simulink model "MalaksModel"  (R2022a)
settings: Solver=FixedStepAuto  StartTime=0.0  StopTime=10  FixedStep=0.001  MaxStep=1  MinStep=5e-4  RelTol=1e-3  EnableMultiTasking=on
values from neighbouring files (symbols this model uses):
  B = 0.00416    [Allan_Param.m]
  b1 = Bf/2    (= 0.776)    [model_10DOF_revised.m]
  b2 = b1    (= 0.776)    [model_10DOF_revised.m]
  b3 = Br/2    (= 0.78)    [model_10DOF_revised.m]
  b4 = b3    (= 0.78)    [model_10DOF_revised.m]
  Beq = 0.0001    [model_10DOF_revised.m]
  Bf = 1.552    [model_10DOF_revised.m]
  cs1 = 4500    [model_10DOF_revised.m]
  cs2 = 4500    [model_10DOF_revised.m]
  cs3 = 11207    [model_10DOF_revised.m]
  dpc = h-hzpc    (= 0.4878144918)    [model_10DOF_revised.m]
  drc = h-hzrc    (= 0.4878144918)    [model_10DOF_revised.m]
  Fs = 100    [Allan_Param.m]
  g = 9.81    [model_10DOF_revised.m]
  hzpc = 0.05    [model_10DOF_revised.m]
  hzrc = 0.05    [model_10DOF_revised.m]
  Ix = 233.072773102 + m*drc^2    (= 616.009936849)    [model_10DOF_revised.m]
  Ix_Iy = Ix -Iy    (= -852.927226898)    [model_10DOF_revised.m]
  Iy = 1086 + m*dpc^2    (= 1468.93716375)    [model_10DOF_revised.m]
  Iy_Iz = Iy -Iz    (= 281.937163747)    [model_10DOF_revised.m]
  Iz = 1187    [model_10DOF_revised.m]
  Iz_Ix = Iz -Ix    (= 570.990063151)    [model_10DOF_revised.m]
  Jeq = 0.00025    [model_10DOF_revised.m]
  K = 1.4e-3    (= 0.0014)    [Allan_Param.m]
  Ka = 0.05    [model_10DOF_revised.m]
  Ke = 0.168    [model_10DOF_revised.m]
  L = 2.72    [model_10DOF_revised.m]
  l1 = 1.12695753    [model_10DOF_revised.m]
  l2 = L-l1    (= 1.59304247)    [model_10DOF_revised.m]
  Leq = 1.5e-3    (= 0.0015)    [model_10DOF_revised.m]
  m = MT-(muf+mur)    (= 1609.23)    [model_10DOF_revised.m]
  mu = 0.8    [model_10DOF_revised.m]
  mu1 = muf/2    (= 49.5)    [model_10DOF_revised.m]
  mu2 = mu1    (= 49.5)    [model_10DOF_revised.m]
  mu3 = mur/2    (= 42)    [model_10DOF_revised.m]
  mu4 = mu3    (= 42)    [model_10DOF_revised.m]
  N = 0.00166667    [Allan_Param.m]
  radius = 40    [path1.m]
  Req = 0.5    [model_10DOF_revised.m]
  ro = 0    [Input.m]
  sw_delta_f = 1    [Input.m]
  Tc = 32    [Allan_Param.m]
  THETAo = 0    [Input.m]
  tpo = cp/6    (= 0.0333333333333)    [Input.m]
  vxo = 10    [Input.m]
  vyo = 0    [Input.m]
  Ws1 = (l2*Ws)/(2*L)    (= 4622.91152767)    [model_10DOF_revised.m]
  x = 0:1:200    [look_ahead.m]    (also in path1.m = x(:))
  Xo = 0    [Input.m]
  y = l_des    [look_ahead.m]    (also in path1.m = zeros(size(x)))
  Yo = 0    [Input.m]
  zu1_0 = -W1/k1t    (= -0.0255425326383)    [model_10DOF_revised.m]
  zu2_0 = -W2/k2t    (= -0.0255425326383)    [model_10DOF_revised.m]
  zu3_0 = -W3/k3t    (= -0.0184119081117)    [model_10DOF_revised.m]
  zu4_0 = -W4/k4t    (= -0.0184119081117)    [model_10DOF_revised.m]
undefined symbols (not defined in the file or in its folder): sw_phi, sw_psi, sw_theta, sw_x, sw_y, sw_zs, sw_zu1, sw_zu2, sw_zu3, sw_zu4
libraries: slpidlib x6, ec_arm_cortex_a_lib x1
(part 1 of 2)
settings Model: Creator=Mohammad Almalak  LastModifiedBy=Mohammad Almalak
settings SolverCC: MaxConsecutiveMinStep=10  PositivePriorityOrder=on
settings OptimizationCC: GainParamInheritBuiltInType=on  DefaultUnderspecifiedDataType=single  EnhancedBackFolding=on  PassReuseOutputArgsAs=Individual arguments  ZeroExternalMemoryAtStartup=off  ZeroInternalMemoryAtStartup=off  MaxStackSize=64  OptimizeBlockOrder=speed  DifferentSizesBufferReuse=on  OptimizationCustomize=off  EfficientTunableParamExpr=on
settings DebuggingCC: ParameterTunabilityLossMsg=error
settings HardwareCC: ProdBitPerPointer=32  ProdBitPerSizeT=32  ProdBitPerPtrDiffT=32  ProdLargestAtomicInteger=Long  ProdLargestAtomicFloat=Double  ProdWordSize=32  ProdHWDeviceType=ARM Compatible->ARM Cortex  TargetBitPerPointer=64  TargetBitPerSizeT=64  TargetBitPerPtrDiffT=64  TargetLongLongMode=on  TargetIntDivRoundTo=Zero  TargetEndianess=LittleEndian  TargetWordSize=64  TargetHWDeviceType=MATLAB Host
settings ModelReferenceCC: ModelReferenceNumInstancesAllowed=Single  ModelReferenceMinAlgLoopOccurrences=on
settings SFSimCC: MATLABDynamicMemAlloc=off
settings RTWCC: SystemTargetFile=ert.tlc  HardwareBoard=BeagleBone Black  TLCOptions="-aInlineSetEventsForThisBaseRateFcn=TLC_FALSE -aSuppressMultiTaskScheduler=TLC_FALSE  -aRateBasedStepFcn=0"  TemplateMakefile=ert_default_tmf  GenerateReport=on  RTWVerbose=off  Toolchain=Linaro Toolchain v4.8  BuildConfiguration=Faster Runs
settings CodeAppCC: ForceParamTrailComments=on  IgnoreCustomStorageClasses=off  MaxIdLength=255  OperatorAnnotations=on  SimulinkDataObjDesc=on  SFDataObjDesc=on  InsertBlockDesc=on
settings ERTTargetCC: SupportContinuousTime=on

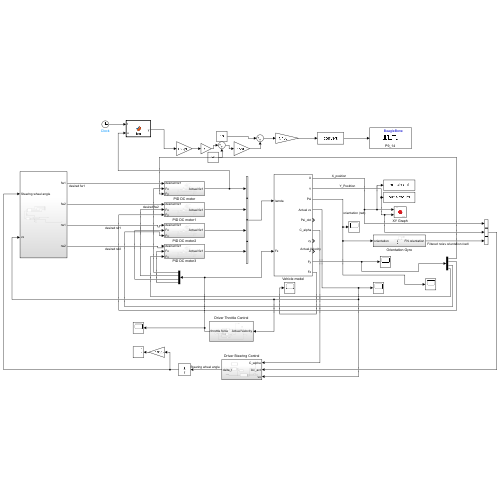
[thumbnail: Simulink's stored preview of the top-level diagram]
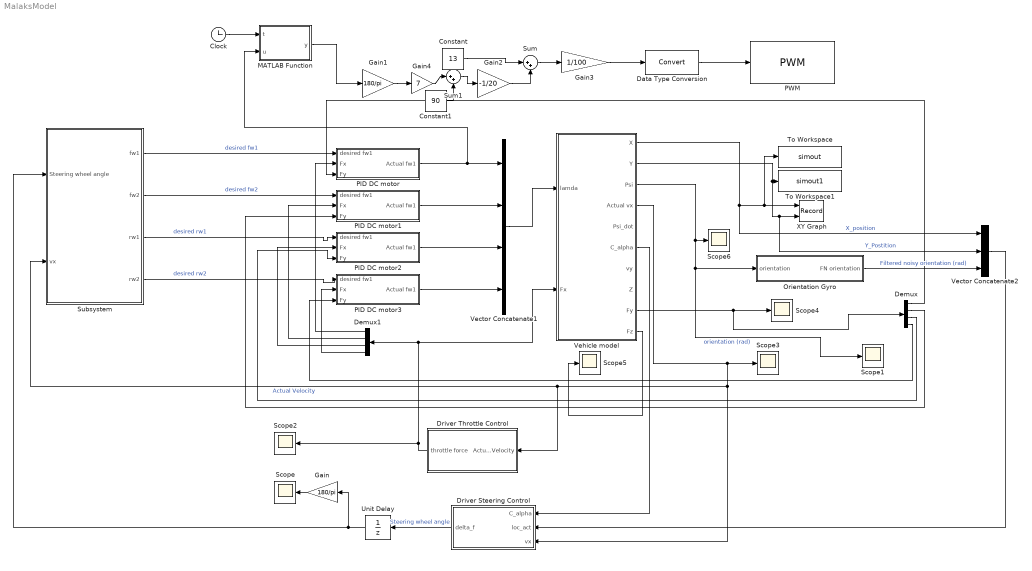
== system MalaksModel ==
  Clock : Clock
  Constant : Constant  Value=13
  Constant1 : Constant  Value=90
  Data Type Conversion : DataTypeConversion  SaturateOnIntegerOverflow=off  RndMeth=Floor
  Demux : Demux
  Demux1 : Demux
  Driver Steering Control : Subsystem
  Driver Throttle Control : Subsystem
  Gain : Gain  Gain=180/pi
  Gain1 : Gain  Gain=180/pi
  Gain2 : Gain  Gain=-1/20
  Gain3 : Gain  Gain=1/100
  Gain4 : Gain  Gain=7
  MATLAB Function : MATLAB Function  TreatAsAtomicUnit=on
  Orientation Gyro : Subsystem
  PID DC motor : Subsystem
  PID DC motor1 : Subsystem
  PID DC motor2 : Subsystem
  PID DC motor3 : Subsystem
  PWM : ec_arm_cortex_a_lib/PWM  board=BeagleBone Black  pin=P9_14  frequency=50  polarity=Positive  blockPlatform=BeagleBone
      settings: SourceProductBaseCode=ECCORTEXA
  Scope{,1..6} (7 alike) : Scope
  Subsystem : Subsystem
  Sum : Sum  Inputs=|++
  Sum1 : Sum  Inputs=|++
  To Workspace : ToWorkspace  VariableName=simout  SaveFormat=Timeseries  SampleTime=-1
  To Workspace1 : ToWorkspace  VariableName=simout1  SaveFormat=Timeseries  SampleTime=-1
  Unit Delay : UnitDelay  SampleTime=-1  HasFrameUpgradeWarning=on
  Vector Concatenate1 : Concatenate  NumInputs=4  ConcatenateDimension=2
  Vector Concatenate2 : Concatenate  NumInputs=3
  Vehicle model : Subsystem
  XY Graph : Record  FileSettingsInternal="{\"entries\":[{\"content\":{\"excelSettings\":{\"content\":{},\"type\":\"Streamout.ExcelSettings\"}},\"type\":\"Streamout.FileSettingStorage\",\"uuid\":\"fef33843-d556-4eb6-a8ea-e7493e2dd152\"}],\"packageUris\":[\"http://schema.mathworks.com/mf0/streamout_blocks/R2020a\"],\"version\":\"1.0\"}"  Layout=[1 1]  SignalsInternal="{\"entries\":[{\"content\":{\"signals\":[{\"content\":{\"blockPath\":[\"MalaksModel/XY Graph\"],\"channel\":[],\"dimensions\":[1],\"domain\":\"MalaksModel/XY Graph\",\"lineColor\":\"#a2142f\",\"plots\":[1],\"port\":1,\"sid\":[\"\"],\"signalID\":362,\"signalName\":\"X_position\"},\"type\":\"RecordBlkView.Signal\",\"uuid\":\"be4ed4d4-a0e0-4c05-83f8-aa9f8cd4aeaf\"},{\"content\":{\"blockPath\":[\"MalaksModel/XY Graph\"],\"channel\":[],\"dimensions\":[1],\"domain\":\"MalaksModel/XY Graph\",\"lineColor\":\"#139fff\",\"plots\":[1],\"port\":2,\"sid\":[\"\"],\"signalID\":366,\"signalName\":\"Y_Postition\"},\"type\":\"RecordBlkView.Signal\",\"uuid\":\"7f74b197-2333-44af-aabe-7eaf48b827cd\"}]},\"type\":\"RecordBlkView.InputSignals\",\"uuid\":\"3425b8f1-97a8-43f9-8de6-0b3d5bc8f21d\"}],\"packageUris\":[\"http://schema.mathworks.com/mf0/streamout_blocks/R2020a\"],\"version\":\"1.0\"}"  VisualizationBindings="{\"xyplotplugin\":{\"info\":[{\"series\":[{\"bindingParametersList\":[{\"parameter\":\"X-Axis\",\"signalID\":362,\"signalName\":\"X_position\"},{\"parameter\":\"Y-Axis\",\"signalID\":366,\"signalName\":\"Y_Postition\"}],\"seriesID\":32300}],\"subplotID\":1}]}}"  CompatibilityTag=XY
  wires:
  Vector Concatenate1/1 -> Vehicle model/1(lamda)
  Vehicle model/3(Psi) -> Scope6/1, Orientation Gyro/1(orientation), Scope1/1  "orientation (rad)"
  Vehicle model/2(Y) -> Vector Concatenate2/2, XY Graph/2, To Workspace1/1  "Y_Postition"
  Vehicle model/1(X) -> Vector Concatenate2/1, To Workspace/1, XY Graph/1  "X_position"
  Vehicle model/4(Actual vx) -> Scope3/1, Driver Steering Control/3(vx), Subsystem/2(vx), Driver Throttle Control/1(Actual Velocity)  "Actual Velocity"
  Vector Concatenate2/1 -> Driver Steering Control/2(loc_act)
  Driver Steering Control/1(delta_f) -> Unit Delay/1  "Steering wheel angle"
  Subsystem/2(fw2) -> PID DC motor1/1(desired fw1)  "desired fw2"
  Subsystem/3(rw1) -> PID DC motor2/1(desired fw1)  "desired rw1"
  Gain/1 -> Scope/1
  Subsystem/4(rw2) -> PID DC motor3/1(desired fw1)  "desired rw2"
  Subsystem/1(fw1) -> PID DC motor/1(desired fw1)  "desired fw1"
  PID DC motor1/1(Actual fw1) -> Vector Concatenate1/2
  PID DC motor2/1(Actual fw1) -> Vector Concatenate1/3
  PID DC motor3/1(Actual fw1) -> Vector Concatenate1/4
  Driver Throttle Control/1(throttle force) -> Scope2/1, Vehicle model/2(Fx), Demux1/1
  Vehicle model/9(Fy) -> Demux/1, Scope4/1
  Demux/1 -> PID DC motor/3(Fy)
  Demux1/1 -> PID DC motor/2(Fx)
  Orientation Gyro/1(FN orientation) -> Vector Concatenate2/3  "Filtered noisy orientation (rad)"
  Demux1/2 -> PID DC motor1/2(Fx)
  Demux1/3 -> PID DC motor2/2(Fx)
  Demux1/4 -> PID DC motor3/2(Fx)
  Demux/2 -> PID DC motor1/3(Fy)
  Demux/3 -> PID DC motor2/3(Fy)
  Demux/4 -> PID DC motor3/3(Fy)
  Vehicle model/10(Fz) -> Scope5/1
  Gain1/1 -> Gain4/1
  Gain2/1 -> Sum/2
  Constant/1 -> Sum/1
  Sum/1 -> Gain3/1
  Data Type Conversion/1 -> PWM/1
  Gain3/1 -> Data Type Conversion/1
  PID DC motor/1(Actual fw1) -> MATLAB Function/2(u), Vector Concatenate1/1
  Vehicle model/6(C_alpha) -> Driver Steering Control/1(C_alpha)
  Unit Delay/1 -> Gain/1, Subsystem/1(Steering wheel angle)
  Gain4/1 -> Sum1/1
  Sum1/1 -> Gain2/1
  Constant1/1 -> Sum1/2
  Clock/1 -> MATLAB Function/1(t)
  MATLAB Function/1(y) -> Gain1/1

== system MalaksModel/Driver Steering Control ==
  C_alpha : Inport  OutDataTypeStr=double
  loc_act : Inport  Port=2  OutDataTypeStr=double
  vx : Inport  Port=3  OutDataTypeStr=double
  FWS Controller : MATLAB Function  TreatAsAtomicUnit=on
  From Workspace : FromWorkspace  VariableName=delta_f
  Subsystem : Subsystem
  Subsystem1 : Subsystem
  delta_f : Outport  OutDataTypeStr=double
  wires:
  FWS Controller/1(ackerman) -> delta_f/1, Subsystem/2(ackerman)
  loc_act/1 -> FWS Controller/1(loc_act)
  C_alpha/1 -> FWS Controller/3(C_alpha)
  From Workspace/1 -> Subsystem/1(In2)
  vx/1 -> FWS Controller/2(vx)

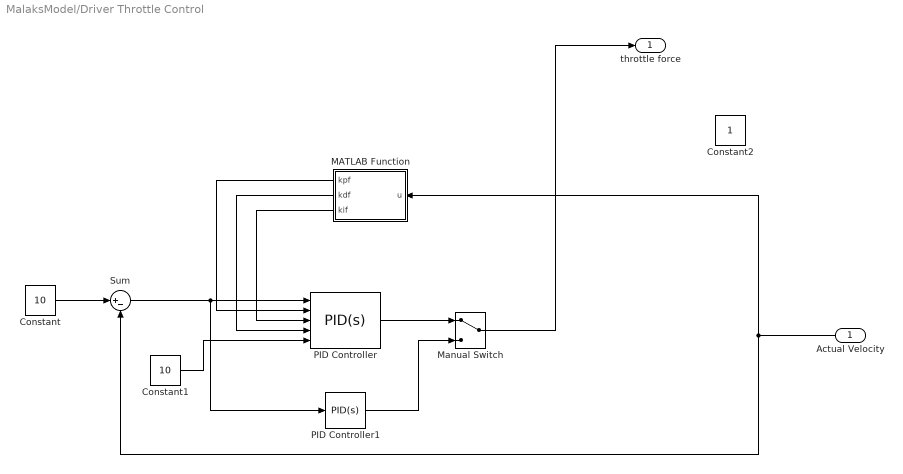
== system MalaksModel/Driver Throttle Control ==
  Actual Velocity : Inport  OutDataTypeStr=double
  Constant : Constant  Value=10
  Constant1 : Constant  Value=10
  Constant2 : Constant
  MATLAB Function : MATLAB Function  TreatAsAtomicUnit=on
  Manual Switch : ManualSwitch
  PID Controller : slpidlib/PID Controller  Controller=PID  Form=Parallel  TimeDomain=Continuous-time  UseExternalTs=off  SampleTime=-1  IntegratorMethod=Forward Euler  FilterMethod=Forward Euler  ControllerParametersSource=external  P=1  I=1  UseKiTs=off  D=0  N=100  UseFilter=on  TunerSelectOption=Transfer Function Based (PID Tuner App)  InitialConditionSource=internal  InitialConditionForIntegrator=0  InitialConditionForFilter=0  DifferentiatorICPrevScaledInput=0  ExternalReset=none  TrackingMode=off  Kt=1  LimitOutput=off  SatLimitsSource=internal  UpperSaturationLimit=inf  LowerSaturationLimit=-inf  LinearizeAsGain=on  AntiWindupMode=none  Kb=1  POutMin=[]  POutMax=[]  IOutMin=[]  IOutMax=[]  DOutMin=[]  DOutMax=[]  NOutMin=[]  NOutMax=[]  SumOutMin=[]  SumOutMax=[]  SaturationOutMin=[]  SaturationOutMax=[]  PParamMin=[]  PParamMax=[]  IParamMin=[]  IParamMax=[]  DParamMin=[]  DParamMax=[]  NParamMin=[]  NParamMax=[]  KbParamMin=[]  KbParamMax=[]  KtParamMin=[]  KtParamMax=[]  KbOutMin=[]  KbOutMax=[]  KtOutMin=[]  KtOutMax=[]  IntegratorOutMin=[]  IntegratorOutMax=[]  FilterOutMin=[]  FilterOutMax=[]  SumI1OutMin=[]  SumI1OutMax=[]  SumI2OutMin=[]  SumI2OutMax=[]  SumI3OutMin=[]  SumI3OutMax=[]  SumI4OutMin=[]  SumI4OutMax=[]  SumDOutMin=[]  SumDOutMax=[]  DifferentiatorOutMin=[]  DifferentiatorOutMax=[]  FilterDiffOutCoefMin=[]  FilterDiffOutCoefMax=[]  ReciprocalOutMin=[]  ReciprocalOutMax=[]  SumDenOutMin=[]  SumDenOutMax=[]  SumNumOutMin=[]  SumNumOutMax=[]  DivideOutMin=[]  DivideOutMax=[]  UdiffTsProdOutMin=[]  UdiffTsProdOutMax=[]  NTsProdOutMin=[]  NTsProdOutMax=[]  UintegralTsProdOutMin=[]  UintegralTsProdOutMax=[]  UngainTsProdOutMin=[]  UngainTsProdOutMax=[]  IntegratorContinuousStateAttributes=''  IntegratorStateMustResolveToSignalObject=off  IntegratorRTWStateStorageClass=Auto  FilterContinuousStateAttributes=''  FilterStateMustResolveToSignalObject=off  FilterRTWStateStorageClass=Auto  ParallelPVariant=ExternalParameters  IdealPVariant=Disabled  IVariant=ExternalParameters  DVariant=ExternalParameters  IntegratorVariant=Continuous  SatVariant=Disabled  AWVariant=Passthrough  PCopyVariant=Disabled  TRVariant=Disabled  FdbkBlocksVariant=Forward  IdealPFdbkVariant=Disabled  SatFdbkVariant=Disabled  DerivativeFilterVariant=ContFilter  NVariant=ExternalParameters  NCopyVariant=Disabled  FilterICVariant=InternalICsFilter  IntegratorICVariant=InternalICs  ExternalResetVariant=Disabled  TRSumVariant=Passthrough  SumFdbkVariant=Disabled  SumVariant=Sum_PID  TsampFilterVariant=InternalTs  TsampNgainVariant=Passthrough  TsampIntegralVariant=Passthrough  ExternalSaturationOutDataTypeStr=Inherit: Same as second input  aMode=0
  PID Controller1 : slpidlib/PID Controller  Controller=PID  Form=Parallel  TimeDomain=Continuous-time  UseExternalTs=off  SampleTime=-1  IntegratorMethod=Forward Euler  FilterMethod=Forward Euler  ControllerParametersSource=internal  P=830.015869772746  I=316.552153422139  UseKiTs=off  D=9.58388407210146  N=238.770606857548  UseFilter=on  TunerSelectOption=Transfer Function Based (PID Tuner App)  InitialConditionSource=internal  InitialConditionForIntegrator=0  InitialConditionForFilter=0  DifferentiatorICPrevScaledInput=0  ExternalReset=none  TrackingMode=off  Kt=1  LimitOutput=off  SatLimitsSource=internal  UpperSaturationLimit=inf  LowerSaturationLimit=-inf  LinearizeAsGain=on  AntiWindupMode=none  Kb=1  POutMin=[]  POutMax=[]  IOutMin=[]  IOutMax=[]  DOutMin=[]  DOutMax=[]  NOutMin=[]  NOutMax=[]  SumOutMin=[]  SumOutMax=[]  SaturationOutMin=[]  SaturationOutMax=[]  PParamMin=[]  PParamMax=[]  IParamMin=[]  IParamMax=[]  DParamMin=[]  DParamMax=[]  NParamMin=[]  NParamMax=[]  KbParamMin=[]  KbParamMax=[]  KtParamMin=[]  KtParamMax=[]  KbOutMin=[]  KbOutMax=[]  KtOutMin=[]  KtOutMax=[]  IntegratorOutMin=[]  IntegratorOutMax=[]  FilterOutMin=[]  FilterOutMax=[]  SumI1OutMin=[]  SumI1OutMax=[]  SumI2OutMin=[]  SumI2OutMax=[]  SumI3OutMin=[]  SumI3OutMax=[]  SumI4OutMin=[]  SumI4OutMax=[]  SumDOutMin=[]  SumDOutMax=[]  DifferentiatorOutMin=[]  DifferentiatorOutMax=[]  FilterDiffOutCoefMin=[]  FilterDiffOutCoefMax=[]  ReciprocalOutMin=[]  ReciprocalOutMax=[]  SumDenOutMin=[]  SumDenOutMax=[]  SumNumOutMin=[]  SumNumOutMax=[]  DivideOutMin=[]  DivideOutMax=[]  UdiffTsProdOutMin=[]  UdiffTsProdOutMax=[]  NTsProdOutMin=[]  NTsProdOutMax=[]  UintegralTsProdOutMin=[]  UintegralTsProdOutMax=[]  UngainTsProdOutMin=[]  UngainTsProdOutMax=[]  IntegratorContinuousStateAttributes=''  IntegratorStateMustResolveToSignalObject=off  IntegratorRTWStateStorageClass=Auto  FilterContinuousStateAttributes=''  FilterStateMustResolveToSignalObject=off  FilterRTWStateStorageClass=Auto  ParallelPVariant=InternalParameters  IdealPVariant=Disabled  IVariant=InternalParameters  DVariant=InternalParameters  IntegratorVariant=Continuous  SatVariant=Disabled  AWVariant=Passthrough  PCopyVariant=Disabled  TRVariant=Disabled  FdbkBlocksVariant=Forward  IdealPFdbkVariant=Disabled  SatFdbkVariant=Disabled  DerivativeFilterVariant=ContFilter  NVariant=InternalParameters  NCopyVariant=Disabled  FilterICVariant=InternalICsFilter  IntegratorICVariant=InternalICs  ExternalResetVariant=Disabled  TRSumVariant=Passthrough  SumFdbkVariant=Disabled  SumVariant=Sum_PID  TsampFilterVariant=InternalTs  TsampNgainVariant=Passthrough  TsampIntegralVariant=Passthrough  ExternalSaturationOutDataTypeStr=Inherit: Same as second input  aMode=0
  Sum : Sum  Inputs=|+-
  throttle force : Outport  OutDataTypeStr=double
  wires:
  MATLAB Function/2(kdf) -> PID Controller/4
  MATLAB Function/3(kif) -> PID Controller/3
  Constant/1 -> Sum/1
  MATLAB Function/1(kpf) -> PID Controller/2
  PID Controller/1 -> Manual Switch/1
  Actual Velocity/1 -> Sum/2, MATLAB Function/1(u)
  Manual Switch/1 -> throttle force/1
  Constant1/1 -> PID Controller/5
  Sum/1 -> PID Controller1/1, PID Controller/1
  PID Controller1/1 -> Manual Switch/2

== system MalaksModel/Orientation Gyro ==
  orientation : Inport  OutDataTypeStr=double
  Allan Noise : Subsystem
  Gain : Gain
  Scope : Scope  NumInputPorts=2
  Sum : Sum  Inputs=|++
  Transfer Fcn : TransferFcn  Numerator=[30]  Denominator=[1 30]
  FN orientation : Outport  OutDataTypeStr=double
  wires:
  Transfer Fcn/1 -> Scope/2, FN orientation/1
  Allan Noise/1(Z) -> Gain/1
  Sum/1 -> Scope/1, Transfer Fcn/1
  orientation/1 -> Sum/1
  Gain/1 -> Sum/2  "rad noise"

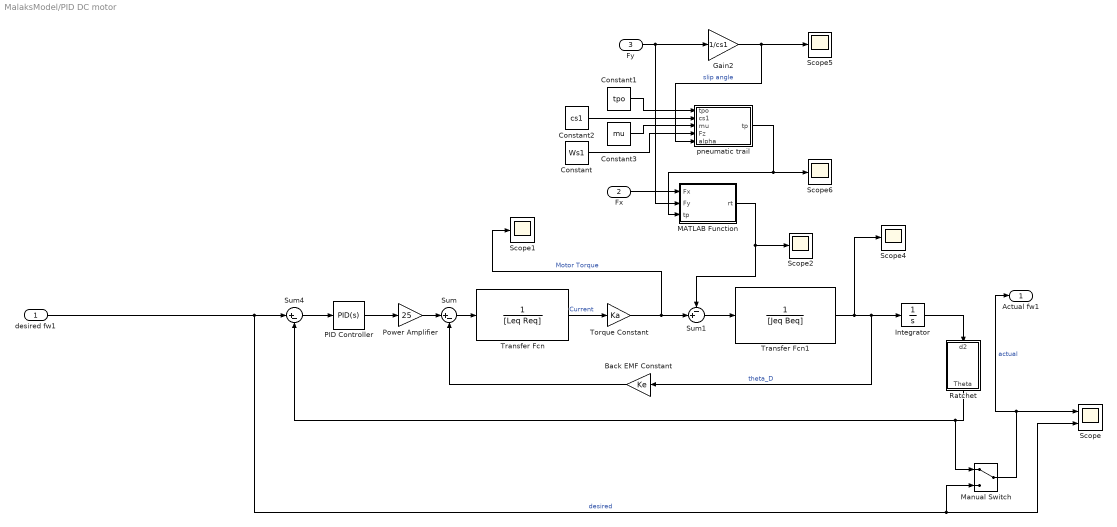
== system MalaksModel/PID DC motor ==
  desired fw1 : Inport  OutDataTypeStr=double
  Fx : Inport  Port=2  OutDataTypeStr=double
  Fy : Inport  Port=3  OutDataTypeStr=double
  Back EMF Constant : Gain  Gain=Ke
  Constant : Constant  Value=Ws1
  Constant1 : Constant  Value=tpo
  Constant2 : Constant  Value=cs1
  Constant3 : Constant  Value=mu
  Gain2 : Gain  Gain=1/cs1
  Integrator : Integrator
  MATLAB Function : MATLAB Function  TreatAsAtomicUnit=on
  Manual Switch : ManualSwitch
  PID Controller : slpidlib/PID Controller  Controller=PID  Form=Parallel  TimeDomain=Continuous-time  UseExternalTs=off  SampleTime=-1  IntegratorMethod=Forward Euler  FilterMethod=Forward Euler  ControllerParametersSource=internal  P=4.49771738027195  I=43.6325510006951  UseKiTs=off  D=-0.104094170262672  N=43.2081582371269  UseFilter=on  TunerSelectOption=Transfer Function Based (PID Tuner App)  InitialConditionSource=internal  InitialConditionForIntegrator=0  InitialConditionForFilter=0  DifferentiatorICPrevScaledInput=0  ExternalReset=none  TrackingMode=off  Kt=1  LimitOutput=off  SatLimitsSource=internal  UpperSaturationLimit=inf  LowerSaturationLimit=-inf  LinearizeAsGain=on  AntiWindupMode=none  Kb=1  POutMin=[]  POutMax=[]  IOutMin=[]  IOutMax=[]  DOutMin=[]  DOutMax=[]  NOutMin=[]  NOutMax=[]  SumOutMin=[]  SumOutMax=[]  SaturationOutMin=[]  SaturationOutMax=[]  PParamMin=[]  PParamMax=[]  IParamMin=[]  IParamMax=[]  DParamMin=[]  DParamMax=[]  NParamMin=[]  NParamMax=[]  KbParamMin=[]  KbParamMax=[]  KtParamMin=[]  KtParamMax=[]  KbOutMin=[]  KbOutMax=[]  KtOutMin=[]  KtOutMax=[]  IntegratorOutMin=[]  IntegratorOutMax=[]  FilterOutMin=[]  FilterOutMax=[]  SumI1OutMin=[]  SumI1OutMax=[]  SumI2OutMin=[]  SumI2OutMax=[]  SumI3OutMin=[]  SumI3OutMax=[]  SumI4OutMin=[]  SumI4OutMax=[]  SumDOutMin=[]  SumDOutMax=[]  DifferentiatorOutMin=[]  DifferentiatorOutMax=[]  FilterDiffOutCoefMin=[]  FilterDiffOutCoefMax=[]  ReciprocalOutMin=[]  ReciprocalOutMax=[]  SumDenOutMin=[]  SumDenOutMax=[]  SumNumOutMin=[]  SumNumOutMax=[]  DivideOutMin=[]  DivideOutMax=[]  UdiffTsProdOutMin=[]  UdiffTsProdOutMax=[]  NTsProdOutMin=[]  NTsProdOutMax=[]  UintegralTsProdOutMin=[]  UintegralTsProdOutMax=[]  UngainTsProdOutMin=[]  UngainTsProdOutMax=[]  IntegratorContinuousStateAttributes=''  IntegratorStateMustResolveToSignalObject=off  IntegratorRTWStateStorageClass=Auto  FilterContinuousStateAttributes=''  FilterStateMustResolveToSignalObject=off  FilterRTWStateStorageClass=Auto  ParallelPVariant=InternalParameters  IdealPVariant=Disabled  IVariant=InternalParameters  DVariant=InternalParameters  IntegratorVariant=Continuous  SatVariant=Disabled  AWVariant=Passthrough  PCopyVariant=Disabled  TRVariant=Disabled  FdbkBlocksVariant=Forward  IdealPFdbkVariant=Disabled  SatFdbkVariant=Disabled  DerivativeFilterVariant=ContFilter  NVariant=InternalParameters  NCopyVariant=Disabled  FilterICVariant=InternalICsFilter  IntegratorICVariant=InternalICs  ExternalResetVariant=Disabled  TRSumVariant=Passthrough  SumFdbkVariant=Disabled  SumVariant=Sum_PID  TsampFilterVariant=InternalTs  TsampNgainVariant=Passthrough  TsampIntegralVariant=Passthrough  ExternalSaturationOutDataTypeStr=Inherit: Same as second input  aMode=0
  Power Amplifier : Gain  Gain=25
  Ratchet : Subsystem
  Scope : Scope  NumInputPorts=2
  Scope{1..2,4..6} (5 alike) : Scope
  Sum : Sum  Inputs=|+-
  Sum1 : Sum  Inputs=-+|
  Sum4 : Sum  Inputs=|+-
  Torque Constant : Gain  Gain=Ka
  Transfer Fcn : TransferFcn  Denominator=[Leq Req]
  Transfer Fcn1 : TransferFcn  Denominator=[Jeq Beq]
  "pneumatic trail " : MATLAB Function  TreatAsAtomicUnit=on
  Actual fw1 : Outport  OutDataTypeStr=double
  wires:
  Transfer Fcn1/1 -> Scope4/1, Integrator/1, Back EMF Constant/1  "theta_D"
  Back EMF Constant/1 -> Sum/2
  Transfer Fcn/1 -> Torque Constant/1  "Current"
  Sum/1 -> Transfer Fcn/1
  desired fw1/1 -> Scope/2, Manual Switch/2, Sum4/1  "desired"
  Manual Switch/1 -> Actual fw1/1, Scope/1  "actual"
  Power Amplifier/1 -> Sum/1
  Sum4/1 -> PID Controller/1
  PID Controller/1 -> Power Amplifier/1
  Fy/1 -> MATLAB Function/2(Fy), Gain2/1
  Gain2/1 -> "pneumatic trail "/5(alpha), Scope5/1  "slip angle"
  Constant1/1 -> "pneumatic trail "/1(tpo)
  Constant2/1 -> "pneumatic trail "/2(cs1)
  Constant3/1 -> "pneumatic trail "/3(mu)
  Constant/1 -> "pneumatic trail "/4(Fz)
  "pneumatic trail "/1(tp) -> MATLAB Function/3(tp), Scope6/1
  Torque Constant/1 -> Scope1/1, Sum1/2  "Motor Torque"
  Sum1/1 -> Transfer Fcn1/1
  MATLAB Function/1(rt) -> Scope2/1, Sum1/1
  Fx/1 -> MATLAB Function/1(Fx)
  Ratchet/1(Theta) -> Manual Switch/1, Sum4/2
  Integrator/1 -> Ratchet/1(d2)

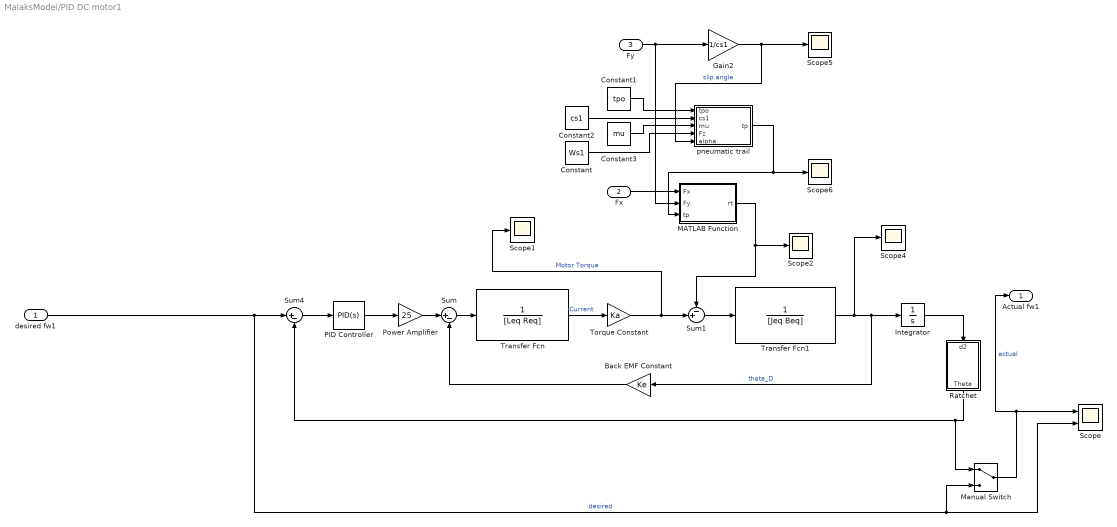
== system MalaksModel/PID DC motor1 ==
  desired fw1 : Inport  OutDataTypeStr=double
  Fx : Inport  Port=2  OutDataTypeStr=double
  Fy : Inport  Port=3  OutDataTypeStr=double
  Back EMF Constant : Gain  Gain=Ke
  Constant : Constant  Value=Ws1
  Constant1 : Constant  Value=tpo
  Constant2 : Constant  Value=cs1
  Constant3 : Constant  Value=mu
  Gain2 : Gain  Gain=1/cs1
  Integrator : Integrator
  MATLAB Function : MATLAB Function  TreatAsAtomicUnit=on
  Manual Switch : ManualSwitch
  PID Controller : slpidlib/PID Controller  Controller=PID  Form=Parallel  TimeDomain=Continuous-time  UseExternalTs=off  SampleTime=-1  IntegratorMethod=Forward Euler  FilterMethod=Forward Euler  ControllerParametersSource=internal  P=4.49771738027195  I=43.6325510006951  UseKiTs=off  D=-0.104094170262672  N=43.2081582371269  UseFilter=on  TunerSelectOption=Transfer Function Based (PID Tuner App)  InitialConditionSource=internal  InitialConditionForIntegrator=0  InitialConditionForFilter=0  DifferentiatorICPrevScaledInput=0  ExternalReset=none  TrackingMode=off  Kt=1  LimitOutput=off  SatLimitsSource=internal  UpperSaturationLimit=inf  LowerSaturationLimit=-inf  LinearizeAsGain=on  AntiWindupMode=none  Kb=1  POutMin=[]  POutMax=[]  IOutMin=[]  IOutMax=[]  DOutMin=[]  DOutMax=[]  NOutMin=[]  NOutMax=[]  SumOutMin=[]  SumOutMax=[]  SaturationOutMin=[]  SaturationOutMax=[]  PParamMin=[]  PParamMax=[]  IParamMin=[]  IParamMax=[]  DParamMin=[]  DParamMax=[]  NParamMin=[]  NParamMax=[]  KbParamMin=[]  KbParamMax=[]  KtParamMin=[]  KtParamMax=[]  KbOutMin=[]  KbOutMax=[]  KtOutMin=[]  KtOutMax=[]  IntegratorOutMin=[]  IntegratorOutMax=[]  FilterOutMin=[]  FilterOutMax=[]  SumI1OutMin=[]  SumI1OutMax=[]  SumI2OutMin=[]  SumI2OutMax=[]  SumI3OutMin=[]  SumI3OutMax=[]  SumI4OutMin=[]  SumI4OutMax=[]  SumDOutMin=[]  SumDOutMax=[]  DifferentiatorOutMin=[]  DifferentiatorOutMax=[]  FilterDiffOutCoefMin=[]  FilterDiffOutCoefMax=[]  ReciprocalOutMin=[]  ReciprocalOutMax=[]  SumDenOutMin=[]  SumDenOutMax=[]  SumNumOutMin=[]  SumNumOutMax=[]  DivideOutMin=[]  DivideOutMax=[]  UdiffTsProdOutMin=[]  UdiffTsProdOutMax=[]  NTsProdOutMin=[]  NTsProdOutMax=[]  UintegralTsProdOutMin=[]  UintegralTsProdOutMax=[]  UngainTsProdOutMin=[]  UngainTsProdOutMax=[]  IntegratorContinuousStateAttributes=''  IntegratorStateMustResolveToSignalObject=off  IntegratorRTWStateStorageClass=Auto  FilterContinuousStateAttributes=''  FilterStateMustResolveToSignalObject=off  FilterRTWStateStorageClass=Auto  ParallelPVariant=InternalParameters  IdealPVariant=Disabled  IVariant=InternalParameters  DVariant=InternalParameters  IntegratorVariant=Continuous  SatVariant=Disabled  AWVariant=Passthrough  PCopyVariant=Disabled  TRVariant=Disabled  FdbkBlocksVariant=Forward  IdealPFdbkVariant=Disabled  SatFdbkVariant=Disabled  DerivativeFilterVariant=ContFilter  NVariant=InternalParameters  NCopyVariant=Disabled  FilterICVariant=InternalICsFilter  IntegratorICVariant=InternalICs  ExternalResetVariant=Disabled  TRSumVariant=Passthrough  SumFdbkVariant=Disabled  SumVariant=Sum_PID  TsampFilterVariant=InternalTs  TsampNgainVariant=Passthrough  TsampIntegralVariant=Passthrough  ExternalSaturationOutDataTypeStr=Inherit: Same as second input  aMode=0
  Power Amplifier : Gain  Gain=25
  Ratchet : Subsystem
  Scope : Scope  NumInputPorts=2
  Scope{1..2,4..6} (5 alike) : Scope
  Sum : Sum  Inputs=|+-
  Sum1 : Sum  Inputs=-+|
  Sum4 : Sum  Inputs=|+-
  Torque Constant : Gain  Gain=Ka
  Transfer Fcn : TransferFcn  Denominator=[Leq Req]
  Transfer Fcn1 : TransferFcn  Denominator=[Jeq Beq]
  "pneumatic trail " : MATLAB Function  TreatAsAtomicUnit=on
  Actual fw1 : Outport  OutDataTypeStr=double
  wires:
  Integrator/1 -> Ratchet/1(d2)
  Ratchet/1(Theta) -> Sum4/2, Manual Switch/1
  Fx/1 -> MATLAB Function/1(Fx)
  MATLAB Function/1(rt) -> Sum1/1, Scope2/1
  Sum1/1 -> Transfer Fcn1/1
  Torque Constant/1 -> Sum1/2, Scope1/1  "Motor Torque"
  "pneumatic trail "/1(tp) -> Scope6/1, MATLAB Function/3(tp)
  Constant/1 -> "pneumatic trail "/4(Fz)
  Constant3/1 -> "pneumatic trail "/3(mu)
  Constant2/1 -> "pneumatic trail "/2(cs1)
  Constant1/1 -> "pneumatic trail "/1(tpo)
  Gain2/1 -> Scope5/1, "pneumatic trail "/5(alpha)  "slip angle"
  Fy/1 -> Gain2/1, MATLAB Function/2(Fy)
  PID Controller/1 -> Power Amplifier/1
  Sum4/1 -> PID Controller/1
  Power Amplifier/1 -> Sum/1
  Manual Switch/1 -> Scope/1, Actual fw1/1  "actual"
  desired fw1/1 -> Sum4/1, Manual Switch/2, Scope/2  "desired"
  Sum/1 -> Transfer Fcn/1
  Transfer Fcn/1 -> Torque Constant/1  "Current"
  Back EMF Constant/1 -> Sum/2
  Transfer Fcn1/1 -> Back EMF Constant/1, Integrator/1, Scope4/1  "theta_D"

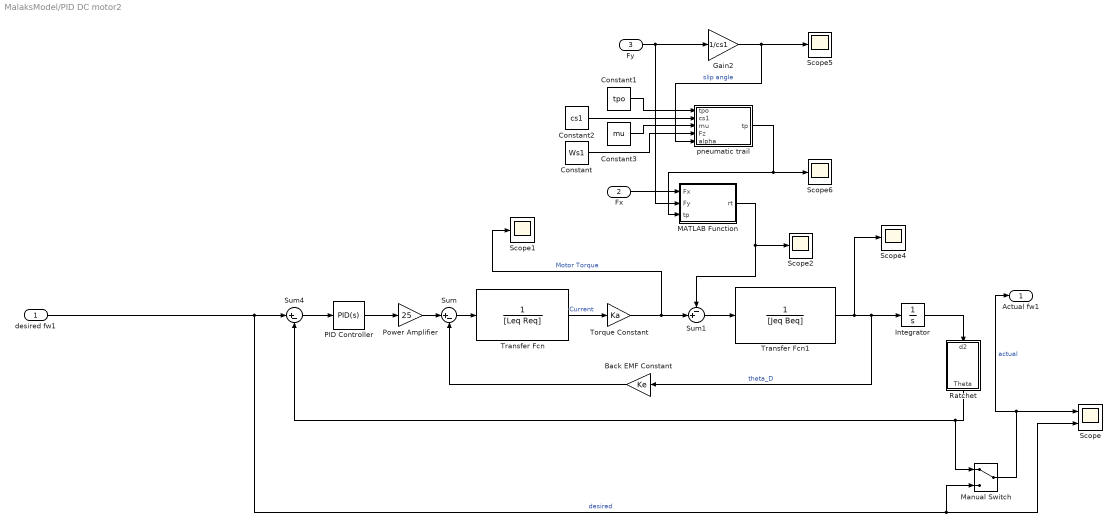
== system MalaksModel/PID DC motor2 ==
  desired fw1 : Inport  OutDataTypeStr=double
  Fx : Inport  Port=2  OutDataTypeStr=double
  Fy : Inport  Port=3  OutDataTypeStr=double
  Back EMF Constant : Gain  Gain=Ke
  Constant : Constant  Value=Ws1
  Constant1 : Constant  Value=tpo
  Constant2 : Constant  Value=cs1
  Constant3 : Constant  Value=mu
  Gain2 : Gain  Gain=1/cs1
  Integrator : Integrator
  MATLAB Function : MATLAB Function  TreatAsAtomicUnit=on
  Manual Switch : ManualSwitch
  PID Controller : slpidlib/PID Controller  Controller=PID  Form=Parallel  TimeDomain=Continuous-time  UseExternalTs=off  SampleTime=-1  IntegratorMethod=Forward Euler  FilterMethod=Forward Euler  ControllerParametersSource=internal  P=4.49771738027195  I=43.6325510006951  UseKiTs=off  D=-0.104094170262672  N=43.2081582371269  UseFilter=on  TunerSelectOption=Transfer Function Based (PID Tuner App)  InitialConditionSource=internal  InitialConditionForIntegrator=0  InitialConditionForFilter=0  DifferentiatorICPrevScaledInput=0  ExternalReset=none  TrackingMode=off  Kt=1  LimitOutput=off  SatLimitsSource=internal  UpperSaturationLimit=inf  LowerSaturationLimit=-inf  LinearizeAsGain=on  AntiWindupMode=none  Kb=1  POutMin=[]  POutMax=[]  IOutMin=[]  IOutMax=[]  DOutMin=[]  DOutMax=[]  NOutMin=[]  NOutMax=[]  SumOutMin=[]  SumOutMax=[]  SaturationOutMin=[]  SaturationOutMax=[]  PParamMin=[]  PParamMax=[]  IParamMin=[]  IParamMax=[]  DParamMin=[]  DParamMax=[]  NParamMin=[]  NParamMax=[]  KbParamMin=[]  KbParamMax=[]  KtParamMin=[]  KtParamMax=[]  KbOutMin=[]  KbOutMax=[]  KtOutMin=[]  KtOutMax=[]  IntegratorOutMin=[]  IntegratorOutMax=[]  FilterOutMin=[]  FilterOutMax=[]  SumI1OutMin=[]  SumI1OutMax=[]  SumI2OutMin=[]  SumI2OutMax=[]  SumI3OutMin=[]  SumI3OutMax=[]  SumI4OutMin=[]  SumI4OutMax=[]  SumDOutMin=[]  SumDOutMax=[]  DifferentiatorOutMin=[]  DifferentiatorOutMax=[]  FilterDiffOutCoefMin=[]  FilterDiffOutCoefMax=[]  ReciprocalOutMin=[]  ReciprocalOutMax=[]  SumDenOutMin=[]  SumDenOutMax=[]  SumNumOutMin=[]  SumNumOutMax=[]  DivideOutMin=[]  DivideOutMax=[]  UdiffTsProdOutMin=[]  UdiffTsProdOutMax=[]  NTsProdOutMin=[]  NTsProdOutMax=[]  UintegralTsProdOutMin=[]  UintegralTsProdOutMax=[]  UngainTsProdOutMin=[]  UngainTsProdOutMax=[]  IntegratorContinuousStateAttributes=''  IntegratorStateMustResolveToSignalObject=off  IntegratorRTWStateStorageClass=Auto  FilterContinuousStateAttributes=''  FilterStateMustResolveToSignalObject=off  FilterRTWStateStorageClass=Auto  ParallelPVariant=InternalParameters  IdealPVariant=Disabled  IVariant=InternalParameters  DVariant=InternalParameters  IntegratorVariant=Continuous  SatVariant=Disabled  AWVariant=Passthrough  PCopyVariant=Disabled  TRVariant=Disabled  FdbkBlocksVariant=Forward  IdealPFdbkVariant=Disabled  SatFdbkVariant=Disabled  DerivativeFilterVariant=ContFilter  NVariant=InternalParameters  NCopyVariant=Disabled  FilterICVariant=InternalICsFilter  IntegratorICVariant=InternalICs  ExternalResetVariant=Disabled  TRSumVariant=Passthrough  SumFdbkVariant=Disabled  SumVariant=Sum_PID  TsampFilterVariant=InternalTs  TsampNgainVariant=Passthrough  TsampIntegralVariant=Passthrough  ExternalSaturationOutDataTypeStr=Inherit: Same as second input  aMode=0
  Power Amplifier : Gain  Gain=25
  Ratchet : Subsystem
  Scope : Scope  NumInputPorts=2
  Scope{1..2,4..6} (5 alike) : Scope
  Sum : Sum  Inputs=|+-
  Sum1 : Sum  Inputs=-+|
  Sum4 : Sum  Inputs=|+-
  Torque Constant : Gain  Gain=Ka
  Transfer Fcn : TransferFcn  Denominator=[Leq Req]
  Transfer Fcn1 : TransferFcn  Denominator=[Jeq Beq]
  "pneumatic trail " : MATLAB Function  TreatAsAtomicUnit=on
  Actual fw1 : Outport  OutDataTypeStr=double
  wires:
  Integrator/1 -> Ratchet/1(d2)
  Ratchet/1(Theta) -> Sum4/2, Manual Switch/1
  Fx/1 -> MATLAB Function/1(Fx)
  MATLAB Function/1(rt) -> Sum1/1, Scope2/1
  Sum1/1 -> Transfer Fcn1/1
  Torque Constant/1 -> Sum1/2, Scope1/1  "Motor Torque"
  "pneumatic trail "/1(tp) -> Scope6/1, MATLAB Function/3(tp)
  Constant/1 -> "pneumatic trail "/4(Fz)
  Constant3/1 -> "pneumatic trail "/3(mu)
  Constant2/1 -> "pneumatic trail "/2(cs1)
  Constant1/1 -> "pneumatic trail "/1(tpo)
  Gain2/1 -> Scope5/1, "pneumatic trail "/5(alpha)  "slip angle"
  Fy/1 -> Gain2/1, MATLAB Function/2(Fy)
  PID Controller/1 -> Power Amplifier/1
  Sum4/1 -> PID Controller/1
  Power Amplifier/1 -> Sum/1
  Manual Switch/1 -> Scope/1, Actual fw1/1  "actual"
  desired fw1/1 -> Sum4/1, Manual Switch/2, Scope/2  "desired"
  Sum/1 -> Transfer Fcn/1
  Transfer Fcn/1 -> Torque Constant/1  "Current"
  Back EMF Constant/1 -> Sum/2
  Transfer Fcn1/1 -> Back EMF Constant/1, Integrator/1, Scope4/1  "theta_D"

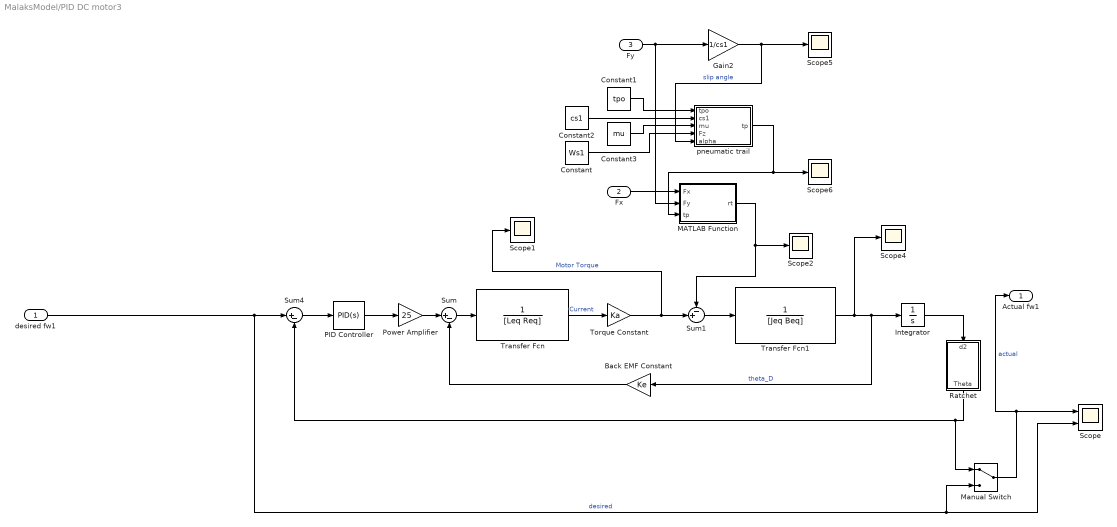
== system MalaksModel/PID DC motor3 ==
  desired fw1 : Inport  OutDataTypeStr=double
  Fx : Inport  Port=2  OutDataTypeStr=double
  Fy : Inport  Port=3  OutDataTypeStr=double
  Back EMF Constant : Gain  Gain=Ke
  Constant : Constant  Value=Ws1
  Constant1 : Constant  Value=tpo
  Constant2 : Constant  Value=cs1
  Constant3 : Constant  Value=mu
  Gain2 : Gain  Gain=1/cs1
  Integrator : Integrator
  MATLAB Function : MATLAB Function  TreatAsAtomicUnit=on
  Manual Switch : ManualSwitch
  PID Controller : slpidlib/PID Controller  Controller=PID  Form=Parallel  TimeDomain=Continuous-time  UseExternalTs=off  SampleTime=-1  IntegratorMethod=Forward Euler  FilterMethod=Forward Euler  ControllerParametersSource=internal  P=4.49771738027195  I=43.6325510006951  UseKiTs=off  D=-0.104094170262672  N=43.2081582371269  UseFilter=on  TunerSelectOption=Transfer Function Based (PID Tuner App)  InitialConditionSource=internal  InitialConditionForIntegrator=0  InitialConditionForFilter=0  DifferentiatorICPrevScaledInput=0  ExternalReset=none  TrackingMode=off  Kt=1  LimitOutput=off  SatLimitsSource=internal  UpperSaturationLimit=inf  LowerSaturationLimit=-inf  LinearizeAsGain=on  AntiWindupMode=none  Kb=1  POutMin=[]  POutMax=[]  IOutMin=[]  IOutMax=[]  DOutMin=[]  DOutMax=[]  NOutMin=[]  NOutMax=[]  SumOutMin=[]  SumOutMax=[]  SaturationOutMin=[]  SaturationOutMax=[]  PParamMin=[]  PParamMax=[]  IParamMin=[]  IParamMax=[]  DParamMin=[]  DParamMax=[]  NParamMin=[]  NParamMax=[]  KbParamMin=[]  KbParamMax=[]  KtParamMin=[]  KtParamMax=[]  KbOutMin=[]  KbOutMax=[]  KtOutMin=[]  KtOutMax=[]  IntegratorOutMin=[]  IntegratorOutMax=[]  FilterOutMin=[]  FilterOutMax=[]  SumI1OutMin=[]  SumI1OutMax=[]  SumI2OutMin=[]  SumI2OutMax=[]  SumI3OutMin=[]  SumI3OutMax=[]  SumI4OutMin=[]  SumI4OutMax=[]  SumDOutMin=[]  SumDOutMax=[]  DifferentiatorOutMin=[]  DifferentiatorOutMax=[]  FilterDiffOutCoefMin=[]  FilterDiffOutCoefMax=[]  ReciprocalOutMin=[]  ReciprocalOutMax=[]  SumDenOutMin=[]  SumDenOutMax=[]  SumNumOutMin=[]  SumNumOutMax=[]  DivideOutMin=[]  DivideOutMax=[]  UdiffTsProdOutMin=[]  UdiffTsProdOutMax=[]  NTsProdOutMin=[]  NTsProdOutMax=[]  UintegralTsProdOutMin=[]  UintegralTsProdOutMax=[]  UngainTsProdOutMin=[]  UngainTsProdOutMax=[]  IntegratorContinuousStateAttributes=''  IntegratorStateMustResolveToSignalObject=off  IntegratorRTWStateStorageClass=Auto  FilterContinuousStateAttributes=''  FilterStateMustResolveToSignalObject=off  FilterRTWStateStorageClass=Auto  ParallelPVariant=InternalParameters  IdealPVariant=Disabled  IVariant=InternalParameters  DVariant=InternalParameters  IntegratorVariant=Continuous  SatVariant=Disabled  AWVariant=Passthrough  PCopyVariant=Disabled  TRVariant=Disabled  FdbkBlocksVariant=Forward  IdealPFdbkVariant=Disabled  SatFdbkVariant=Disabled  DerivativeFilterVariant=ContFilter  NVariant=InternalParameters  NCopyVariant=Disabled  FilterICVariant=InternalICsFilter  IntegratorICVariant=InternalICs  ExternalResetVariant=Disabled  TRSumVariant=Passthrough  SumFdbkVariant=Disabled  SumVariant=Sum_PID  TsampFilterVariant=InternalTs  TsampNgainVariant=Passthrough  TsampIntegralVariant=Passthrough  ExternalSaturationOutDataTypeStr=Inherit: Same as second input  aMode=0
  Power Amplifier : Gain  Gain=25
  Ratchet : Subsystem
  Scope : Scope  NumInputPorts=2
  Scope{1..2,4..6} (5 alike) : Scope
  Sum : Sum  Inputs=|+-
  Sum1 : Sum  Inputs=-+|
  Sum4 : Sum  Inputs=|+-
  Torque Constant : Gain  Gain=Ka
  Transfer Fcn : TransferFcn  Denominator=[Leq Req]
  Transfer Fcn1 : TransferFcn  Denominator=[Jeq Beq]
  "pneumatic trail " : MATLAB Function  TreatAsAtomicUnit=on
  Actual fw1 : Outport  OutDataTypeStr=double
  wires:
  Integrator/1 -> Ratchet/1(d2)
  Ratchet/1(Theta) -> Sum4/2, Manual Switch/1
  Fx/1 -> MATLAB Function/1(Fx)
  MATLAB Function/1(rt) -> Sum1/1, Scope2/1
  Sum1/1 -> Transfer Fcn1/1
  Torque Constant/1 -> Sum1/2, Scope1/1  "Motor Torque"
  "pneumatic trail "/1(tp) -> Scope6/1, MATLAB Function/3(tp)
  Constant/1 -> "pneumatic trail "/4(Fz)
  Constant3/1 -> "pneumatic trail "/3(mu)
  Constant2/1 -> "pneumatic trail "/2(cs1)
  Constant1/1 -> "pneumatic trail "/1(tpo)
  Gain2/1 -> Scope5/1, "pneumatic trail "/5(alpha)  "slip angle"
  Fy/1 -> Gain2/1, MATLAB Function/2(Fy)
  PID Controller/1 -> Power Amplifier/1
  Sum4/1 -> PID Controller/1
  Power Amplifier/1 -> Sum/1
  Manual Switch/1 -> Scope/1, Actual fw1/1  "actual"
  desired fw1/1 -> Sum4/1, Manual Switch/2, Scope/2  "desired"
  Sum/1 -> Transfer Fcn/1
  Transfer Fcn/1 -> Torque Constant/1  "Current"
  Back EMF Constant/1 -> Sum/2
  Transfer Fcn1/1 -> Back EMF Constant/1, Integrator/1, Scope4/1  "theta_D"

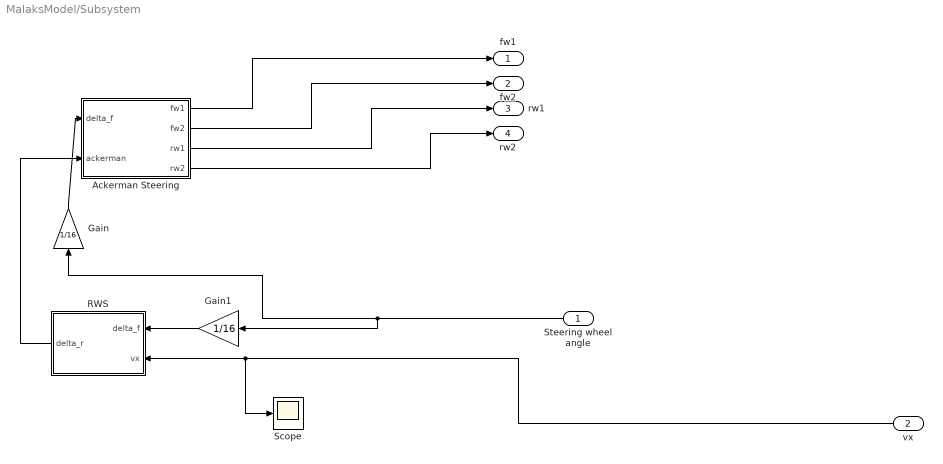
== system MalaksModel/Subsystem ==
  Steering wheel angle : Inport  OutDataTypeStr=double
  vx : Inport  Port=2  OutDataTypeStr=double
  Ackerman Steering : Subsystem
  Gain : Gain  Gain=1/16
  Gain1 : Gain  Gain=1/16
  RWS : Subsystem
  Scope : Scope
  fw1 : Outport  OutDataTypeStr=double
  fw2 : Outport  Port=2  OutDataTypeStr=double
  rw1 : Outport  Port=3  OutDataTypeStr=double
  rw2 : Outport  Port=4  OutDataTypeStr=double
  wires:
  Ackerman Steering/4(rw2) -> rw2/1
  Gain/1 -> Ackerman Steering/1(delta_f)
  Gain1/1 -> RWS/1(delta_f)
  Steering wheel angle/1 -> Gain/1, Gain1/1
  RWS/1(delta_r) -> Ackerman Steering/2(ackerman)
  Ackerman Steering/1(fw1) -> fw1/1
  Ackerman Steering/3(rw1) -> rw1/1
  Ackerman Steering/2(fw2) -> fw2/1
  vx/1 -> Scope/1, RWS/2(vx)

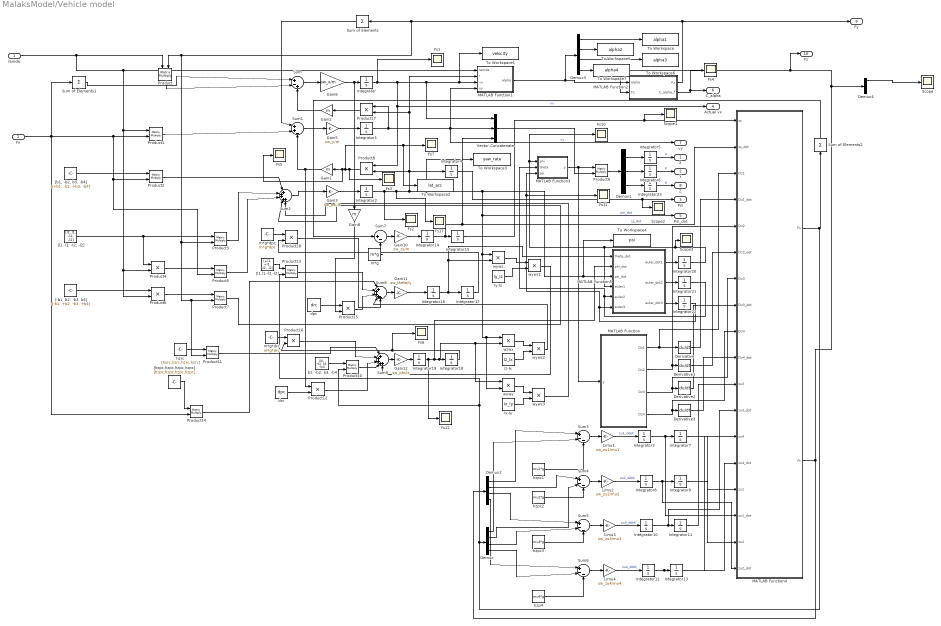
== system MalaksModel/Vehicle model ==
  lamda : Inport  OutDataTypeStr=double
  Fx : Inport  Port=2  OutDataTypeStr=double
  1/mu2 : Gain  Gain=sw_zu2/mu2
  1/mu3 : Gain  Gain=sw_zu3/mu3
  1/mu4 : Gain  Gain=sw_zu4/mu4
  Demux{,2..4} (4 alike) : Demux
  Demux1 : Demux  Outputs=3
      settings: DisplayOption=none
  Derivative{,1..3} (4 alike) : Derivative
  Fs{1..7,10..12,17} (11 alike) : Scope
  Gain1 : Gain  Gain=m
  Gain10 : Gain  Gain=sw_zs/m
  Gain11 : Gain  Gain=sw_theta/Iy
  Gain12 : Gain  Gain=sw_phi/Ix
  Gain2 : Gain  Gain=m
  Gain3 : Gain  Gain=sw_psi/Iz
  Gain5 : Gain  Gain=sw_y/m
  Gain6 : Gain  Gain=sw_x/m
  Gain8 : Gain  Gain=m
  Integrator : Integrator  InitialCondition=vxo
  Integrator1 : Integrator  InitialCondition=vyo
  Integrator{3,8,10,12,14,16..22} (12 alike) : Integrator
  Integrator11 : Integrator  InitialCondition=zu3_0
  Integrator13 : Integrator  InitialCondition=zu4_0
  Integrator15 : Integrator  InitialCondition=-0.058
  Integrator2 : Integrator  InitialCondition=ro
  Integrator23 : Integrator  InitialCondition=Yo
  Integrator4 : Integrator  InitialCondition=THETAo
  Integrator5 : Integrator  InitialCondition=Xo
  Integrator6 : Integrator  InitialCondition=Yo
  Integrator7 : Integrator  InitialCondition=zu1_0
  Integrator9 : Integrator  InitialCondition=zu2_0
  Ix-Iy : Constant  Value=Ix_Iy  VectorParams1D=off
  Iy-Iz : Constant  Value=Iy_Iz  VectorParams1D=off
  Iz-Ix : Constant  Value=Iz_Ix  VectorParams1D=off
  MATLAB Function : MATLAB Function  TreatAsAtomicUnit=on
  MATLAB Function1 : MATLAB Function  TreatAsAtomicUnit=on
  MATLAB Function2 : MATLAB Function  TreatAsAtomicUnit=on
  MATLAB Function3 : MATLAB Function  TreatAsAtomicUnit=on
  MATLAB Function4 : MATLAB Function  TreatAsAtomicUnit=on
  MATLAB Function5 : MATLAB Function  TreatAsAtomicUnit=on
  Product{,1..3,5,7,9..11,13..14} (11 alike) : Product  Multiplication=Matrix(*)
  Product{4,6,8,12,15..18} (8 alike) : Product
  Scope{,1..3} (4 alike) : Scope
  Sum : Sum  Inputs=|+-+
  Sum of Elements : Sum  Inputs=+
  Sum of Elements1 : Sum  Inputs=+
  Sum of Elements2 : Sum  Inputs=+
  Sum1 : Sum  Inputs=|++-
  Sum2 : Sum  Inputs=|+++++
  Sum{3..6} (4 alike) : Sum  Inputs=|+--
  Sum7 : Sum  Inputs=|+-
  Sum8 : Sum  Inputs=|+++++
  Sum9 : Sum  Inputs=|+++++
  To Workspace : ToWorkspace  VariableName=alpha1  SaveFormat=Timeseries  SampleTime=-1
      settings: Save2DSignal=2-D array (concatenate along first dimension)
  To Workspace1 : ToWorkspace  VariableName=velocity  SaveFormat=Timeseries  SampleTime=-1
  To Workspace2 : ToWorkspace  VariableName=lat_acc  SaveFormat=Timeseries  SampleTime=-1
  To Workspace3 : ToWorkspace  VariableName=yaw_rate  SaveFormat=Timeseries  SampleTime=-1
  To Workspace4 : ToWorkspace  VariableName=psi  SaveFormat=Timeseries  SampleTime=-1
  To Workspace5 : ToWorkspace  VariableName=alpha2  SaveFormat=Timeseries  SampleTime=-1
      settings: Save2DSignal=2-D array (concatenate along first dimension)
  To Workspace6 : ToWorkspace  VariableName=alpha3  SaveFormat=Timeseries  SampleTime=-1
      settings: Save2DSignal=2-D array (concatenate along first dimension)
  To Workspace7 : ToWorkspace  VariableName=alpha4  SaveFormat=Timeseries  SampleTime=-1
      settings: Save2DSignal=2-D array (concatenate along first dimension)
  Vector Concatenate : Concatenate  NumInputs=3
  "[-b1, b2, -b3, b4]" : Constant  Value=[-b1, +b2, -b3, +b4]  VectorParams1D=off
  "[b1, -b2, b3, -b4]" : Constant  Value=[+b1, -b2, +b3, -b4]  VectorParams1D=off
  "[hzpc,hzpc,hzpc,hzpc]" : Constant  Value=[hzpc,hzpc,hzpc,hzpc]  VectorParams1D=off
  "[l1, l1, -l2, -l2]" : Constant  Value=[l1, l1, -l2, -l2]  VectorParams1D=off
  "[l1,l1,-l2,-l2]" : Constant  Value=[+l1, +l1, -l2, -l2]  VectorParams1D=off
  `1/mu1 : Gain  Gain=sw_zu1/mu1
  "b1, -b2, b3, -b4" : Constant  Value=[b1, -b2, b3, -b4]  VectorParams1D=off
  dpc : Constant  Value=drc  VectorParams1D=off
  drc : Constant  Value=dpc  VectorParams1D=off
  hzp4 : Constant  Value=mu4*g  VectorParams1D=off
  hzpc1 : Constant  Value=mu1*g  VectorParams1D=off
  hzpc2 : Constant  Value=mu2*g  VectorParams1D=off
  hzpc3 : Constant  Value=mu3*g  VectorParams1D=off
  hzrc : Constant  Value=[hzrc,hzrc,hzrc,hzrc]  VectorParams1D=off
  m*g : Constant  Value=m*g  VectorParams1D=off
  m*g*dpc : Constant  Value=m*g*dpc  VectorParams1D=off
  m*g*drc : Constant  Value=m*g*drc  VectorParams1D=off
  wxwy : Product
  wywz{,1..3} (4 alike) : Product
  wzwx : Product
  X : Outport  OutDataTypeStr=double
  Y : Outport  Port=2  OutDataTypeStr=double
  Psi : Outport  Port=3  OutDataTypeStr=double
  Actual vx : Outport  Port=4  OutDataTypeStr=double
  Psi_dot : Outport  Port=5  OutDataTypeStr=double
  C_alpha : Outport  Port=6  OutDataTypeStr=double
  vy : Outport  Port=7  OutDataTypeStr=double
  Z : Outport  Port=8  OutDataTypeStr=double
  Fy : Outport  Port=9  OutDataTypeStr=double
  Fz : Outport  Port=10  OutDataTypeStr=double
  wires:
  Product11/1 -> Sum9/1
  wywz1/1 -> Sum9/5
  Demux3/4 -> To Workspace7/1
  Demux3/3 -> To Workspace6/1
  Demux3/2 -> To Workspace5/1
  Demux3/1 -> To Workspace/1
  Product/1 -> Sum/2
  Gain2/1 -> Sum/3
  MATLAB Function1/1(alpha) -> Demux3/1, MATLAB Function2/1(alpha)
  Integrator11/1 -> MATLAB Function4/11(zu3)
  Integrator13/1 -> MATLAB Function4/13(zu4)
  Integrator7/1 -> MATLAB Function4/15(zu1)
  Integrator4/1 -> Scope2/1, Psi/1
  Product18/1 -> Sum8/5
  Integrator17/1 -> Product18/2
  m*g*dpc/1 -> Product18/1
  Product17/1 -> Gain2/1
  Derivative3/1 -> MATLAB Function4/10(Dz4_dot)
  Derivative2/1 -> MATLAB Function4/8(Dz3_dot)
  Derivative1/1 -> MATLAB Function4/6(Dz2_dot)
  Derivative/1 -> MATLAB Function4/4(Dz1_dot)
  MATLAB Function/2(Dz2) -> Derivative1/1, MATLAB Function4/5(Dz2)
  MATLAB Function/4(Dz4) -> Derivative3/1, MATLAB Function4/9(Dz4)
  MATLAB Function/3(Dz3) -> Derivative2/1, MATLAB Function4/7(Dz3)
  MATLAB Function/1(Dz1) -> Derivative/1, MATLAB Function4/3(Dz1)
  Demux1/3 -> Integrator23/1
  Integrator23/1 -> Z/1  "p"
  Sum of Elements2/1 -> Sum7/1
  MATLAB Function4/2(Ft) -> Demux2/1, Demux4/1, Fz/1, MATLAB Function2/2(Fz)
  MATLAB Function4/1(Fs) -> Demux/1, Product13/2, Product10/2, Sum of Elements2/1
  Integrator9/1 -> MATLAB Function4/17(zu2)
  Integrator15/1 -> Scope1/1, MATLAB Function4/1(zs)
  Integrator22/1 -> MATLAB Function5/6(euler3), Fs11/1, MATLAB Function3/3(psi)
  Integrator21/1 -> MATLAB Function5/5(euler2), MATLAB Function3/2(theta)
  MATLAB Function5/3(euler_dot3) -> Integrator22/1
  MATLAB Function5/2(euler_dot2) -> Integrator21/1
  MATLAB Function5/1(euler_dot1) -> Integrator20/1
  Integrator20/1 -> Scope3/1, MATLAB Function5/4(euler1), MATLAB Function3/1(phi), Fs10/1
  wywz3/1 -> Sum2/5
  wywz2/1 -> Sum8/4
  Iy-Iz/1 -> wywz1/2
  wywz/1 -> wywz1/1
  Iz-Ix/1 -> wywz2/2
  wzwx/1 -> wywz2/1
  Ix-Iy/1 -> wywz3/2
  wxwy/1 -> wywz3/1
  m*g/1 -> Sum7/2
  hzpc1/1 -> Sum3/3
  hzpc2/1 -> Sum4/3
  hzpc3/1 -> Sum5/3
  hzp4/1 -> Sum6/3
  Demux/4 -> Sum6/2
  Demux/3 -> Sum5/2
  Demux/2 -> Sum4/2
  Demux/1 -> Sum3/2
  Demux2/4 -> Sum6/1
  Demux2/3 -> Sum5/1
  Demux2/2 -> Sum4/1
  Demux2/1 -> Sum3/1
  Gain12/1 -> Integrator19/1
  Sum9/1 -> Gain12/1
  Gain11/1 -> Integrator16/1
  Sum8/1 -> Gain11/1
  Gain10/1 -> Integrator14/1
  Sum7/1 -> Gain10/1
  Product15/1 -> Sum8/3
  Gain8/1 -> Product15/2
  dpc/1 -> Product15/1
  Product13/1 -> Sum8/2
  "[l1,l1,-l2,-l2]"/1 -> Product13/1
  Product14/1 -> Sum8/1
  Product16/1 -> Sum9/2
  m*g*drc/1 -> Product16/1
  Product12/1 -> Sum9/3
  drc/1 -> Product12/2
  Product10/1 -> Sum9/4
  "b1, -b2, b3, -b4"/1 -> Product10/1
  Integrator18/1 -> Product16/2, Fs6/1
  Integrator19/1 -> Integrator18/1, wzwx/2, wxwy/1, MATLAB Function5/2(phi_dot), Fs12/1
  Integrator16/1 -> Integrator17/1, wywz/2, MATLAB Function5/1(theta_dot)
  Integrator14/1 -> Integrator15/1, MATLAB Function4/2(zs_dot), Vector Concatenate/3  "zs_dot"
  Sum6/1 -> 1/mu4/1
  1/mu4/1 -> Integrator12/1  "zu4_ddot"
  Integrator12/1 -> Integrator13/1, MATLAB Function4/14(zu4_dot)
  Sum5/1 -> 1/mu3/1
  1/mu3/1 -> Integrator10/1  "zu3_ddot"
  Integrator10/1 -> Integrator11/1, MATLAB Function4/12(zu3_dot)
  Sum4/1 -> 1/mu2/1
  1/mu2/1 -> Integrator8/1  "zu2_ddot"
  Integrator8/1 -> Integrator9/1, MATLAB Function4/18(zu2_dot)
  Integrator3/1 -> Integrator7/1, MATLAB Function4/16(zu1_dot)
  `1/mu1/1 -> Integrator3/1  "zu1_ddot"
  Sum3/1 -> `1/mu1/1
  "[hzpc,hzpc,hzpc,hzpc]"/1 -> Product14/1
  hzrc/1 -> Product11/1
  Gain1/1 -> Product12/1, Sum1/3
  Gain5/1 -> Integrator1/1
  Sum1/1 -> Gain5/1
  Sum/1 -> Gain6/1
  Gain6/1 -> Gain8/1, Integrator/1
  Sum2/1 -> Gain3/1
  Gain3/1 -> Integrator2/1
  MATLAB Function2/2(C_alpha_f) -> C_alpha/1, Fs4/1
  lamda/1 -> MATLAB Function1/1(lamda), Product1/1, Product6/2, Product4/2, Product/1
  "[-b1, b2, -b3, b4]"/1 -> Product6/1
  Integrator5/1 -> X/1  "p"
  Sum of Elements/1 -> Sum1/1
  "[b1, -b2, b3, -b4]"/1 -> Product2/1
  Product1/1 -> Sum1/2
  Demux1/2 -> Integrator6/1
  MATLAB Function3/1(y) -> MATLAB Function/1(y), Product9/1
  Demux1/1 -> Integrator5/1
  Vector Concatenate/1 -> Product9/2
  Product7/1 -> Sum2/4
  Integrator6/1 -> Y/1  "p"
  Product2/1 -> Sum2/1
  Integrator/1 -> Actual vx/1, Product8/1, Vector Concatenate/1, MATLAB Function1/3(vx), To Workspace1/1, Fs1/1  "vx"
  Product8/1 -> Gain1/1, Fs5/1, To Workspace2/1, Fs7/1, Fs3/1
  Sum of Elements1/1 -> Sum/1
  Product6/1 -> Product7/1
  MATLAB Function2/1(Fy) -> Product/2, Product3/2, Product11/2, Product7/2, Sum of Elements/1, Fy/1
  Integrator2/1 -> Integrator4/1, Product8/2, Product17/2, MATLAB Function1/2(r), Psi_dot/1, wywz/1, wzwx/1, wxwy/2, MATLAB Function5/3(psi_dot), To Workspace4/1, To Workspace3/1, Fs17/1, Fs2/1  "psi_dot"
  Product3/1 -> Sum2/2
  Product4/1 -> Product5/1
  Product9/1 -> Demux1/1
  Product5/1 -> Sum2/3
  "[l1, l1, -l2, -l2]"/1 -> Product3/1, Product4/1
  Fx/1 -> Sum of Elements1/1, Product1/2, Product2/2, Product5/2, Product14/2
  Integrator1/1 -> MATLAB Function1/4(vy), vy/1, Vector Concatenate/2, Product17/1  "vy"
  Demux4/1 -> Scope/1

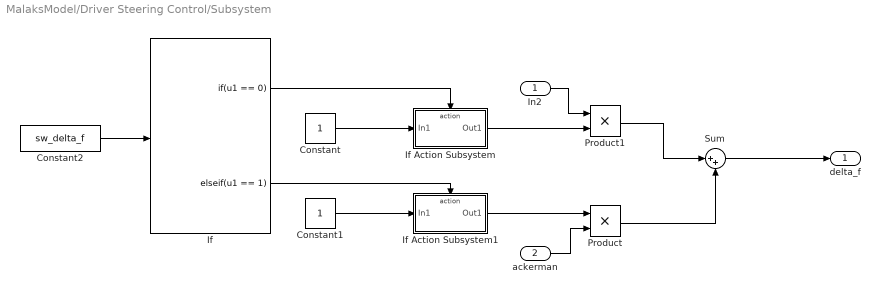
== system MalaksModel/Driver Steering Control/Subsystem ==
  In2 : Inport
  ackerman : Inport  Port=2
  Constant : Constant
  Constant1 : Constant
  Constant2 : Constant  Value=sw_delta_f
  If : If  IfExpression=u1 == 0  ElseIfExpressions=u1 == 1  ShowElse=off
  If Action Subsystem : Subsystem  TreatAsAtomicUnit=on
  If Action Subsystem1 : Subsystem  TreatAsAtomicUnit=on
  Product : Product
  Product1 : Product
  Sum : Sum  Inputs=|++
  delta_f : Outport
  wires:
  Sum/1 -> delta_f/1
  Product/1 -> Sum/2
  Product1/1 -> Sum/1
  ackerman/1 -> Product/2
  In2/1 -> Product1/1
  If Action Subsystem1/1(Out1) -> Product/1
  Constant1/1 -> If Action Subsystem1/1(In1)
  Constant/1 -> If Action Subsystem/1(In1)
  If Action Subsystem/1(Out1) -> Product1/2
  If/2 -> If Action Subsystem1/Action
  If/1 -> If Action Subsystem/Action
  Constant2/1 -> If/1

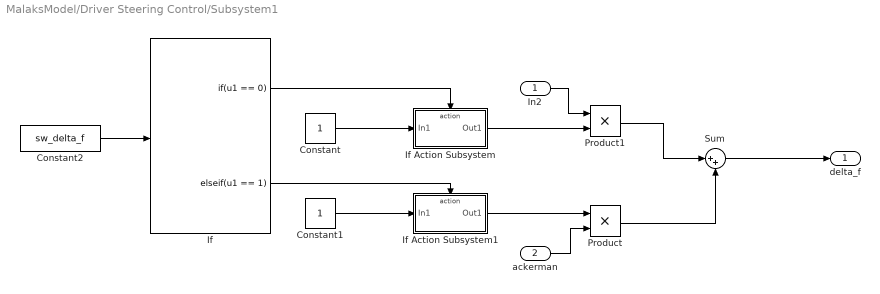
== system MalaksModel/Driver Steering Control/Subsystem1 ==
  In2 : Inport
  ackerman : Inport  Port=2
  Constant : Constant
  Constant1 : Constant
  Constant2 : Constant  Value=sw_delta_f
  If : If  IfExpression=u1 == 0  ElseIfExpressions=u1 == 1  ShowElse=off
  If Action Subsystem : Subsystem  TreatAsAtomicUnit=on
  If Action Subsystem1 : Subsystem  TreatAsAtomicUnit=on
  Product : Product
  Product1 : Product
  Sum : Sum  Inputs=|++
  delta_f : Outport
  wires:
  Constant2/1 -> If/1
  If/1 -> If Action Subsystem/Action
  If/2 -> If Action Subsystem1/Action
  If Action Subsystem/1(Out1) -> Product1/2
  Constant/1 -> If Action Subsystem/1(In1)
  Constant1/1 -> If Action Subsystem1/1(In1)
  If Action Subsystem1/1(Out1) -> Product/1
  In2/1 -> Product1/1
  ackerman/1 -> Product/2
  Product1/1 -> Sum/1
  Product/1 -> Sum/2
  Sum/1 -> delta_f/1

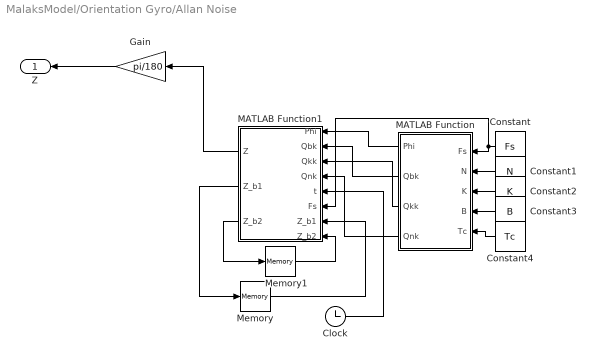
== system MalaksModel/Orientation Gyro/Allan Noise ==
  Clock : Clock
  Constant : Constant  Value=Fs
  Constant1 : Constant  Value=N
  Constant2 : Constant  Value=K
  Constant3 : Constant  Value=B
  Constant4 : Constant  Value=Tc
  Gain : Gain  Gain=pi/180
  MATLAB Function : MATLAB Function  TreatAsAtomicUnit=on
  MATLAB Function1 : MATLAB Function  TreatAsAtomicUnit=on
  Memory : Memory  InheritSampleTime=on
  Memory1 : Memory  InheritSampleTime=on
  Z : Outport  OutDataTypeStr=double
  wires:
  MATLAB Function/1(Phi) -> MATLAB Function1/1(Phi)
  Memory/1 -> MATLAB Function1/7("Z_b1 ")
  MATLAB Function1/2(Z_b1) -> Memory/1
  MATLAB Function/2(Qbk) -> MATLAB Function1/2(Qbk)
  Constant2/1 -> MATLAB Function/3(K)
  Clock/1 -> MATLAB Function1/5(t)
  Constant3/1 -> MATLAB Function/4(B)
  Memory1/1 -> MATLAB Function1/8("Z_b2 ")
  MATLAB Function1/3(Z_b2) -> Memory1/1
  Constant1/1 -> MATLAB Function/2(N)
  MATLAB Function/3(Qkk) -> MATLAB Function1/3(Qkk)
  MATLAB Function/4(Qnk) -> MATLAB Function1/4(Qnk)
  Constant/1 -> MATLAB Function1/6(Fs), MATLAB Function/1(Fs)
  Constant4/1 -> MATLAB Function/5(Tc)
  MATLAB Function1/1(Z) -> Gain/1
  Gain/1 -> Z/1

== system MalaksModel/PID DC motor/Ratchet ==
  d2 : Inport  OutDataTypeStr=double
  Memory3 : Memory
  Memory4 : Memory
  Ratchet : MATLAB Function  TreatAsAtomicUnit=on
  Switch : MATLAB Function  TreatAsAtomicUnit=on
  Theta : Outport  OutDataTypeStr=double
  wires:
  Switch/1(y) -> Ratchet/3(s)
  Ratchet/1(y) -> Theta/1, Memory4/1  "Theta"
  Memory4/1 -> Ratchet/2(d1)
  Switch/2(d) -> Memory3/1
  d2/1 -> Switch/1(d2), Ratchet/1(d2)
  Memory3/1 -> Switch/2(d1)
